simulink library "posAug_cl_old"  (R2022a)
settings: Solver=VariableStepAuto  StartTime=0.0  StopTime=10.0  RelTol=1e-3
undefined symbols (not defined in the file): aoaStart, elevSet, elevStart, env, FLIGHTCONTROLLER, fltCtrl, initializeBussesFromBlock, intSat, pathLaps, pathLapsYaw, posAug, rollAmp, rollFreq, rollPhase, sEstim, slfExitTime, thetaIGain, thetaPGain, vhcl, yawAmp, yawFreq, yawPhase
libraries: slpidlib x10, simulink x5, posAug_cl_new x4, velocityAngle_ul x4, dspsigops x3, pathFollowingCtrlAoATurb_cl x1, pathFollowingCtrlAoATurbCoef_cl x1, courseFollowLookAhead_cl x1, ctrlAllocMatrix3CompCoef_cl x1, eulAng2RotMat_ul x1, $bdroot x1, angleBtw2Vecs_ul x1
(part 3 of 3)

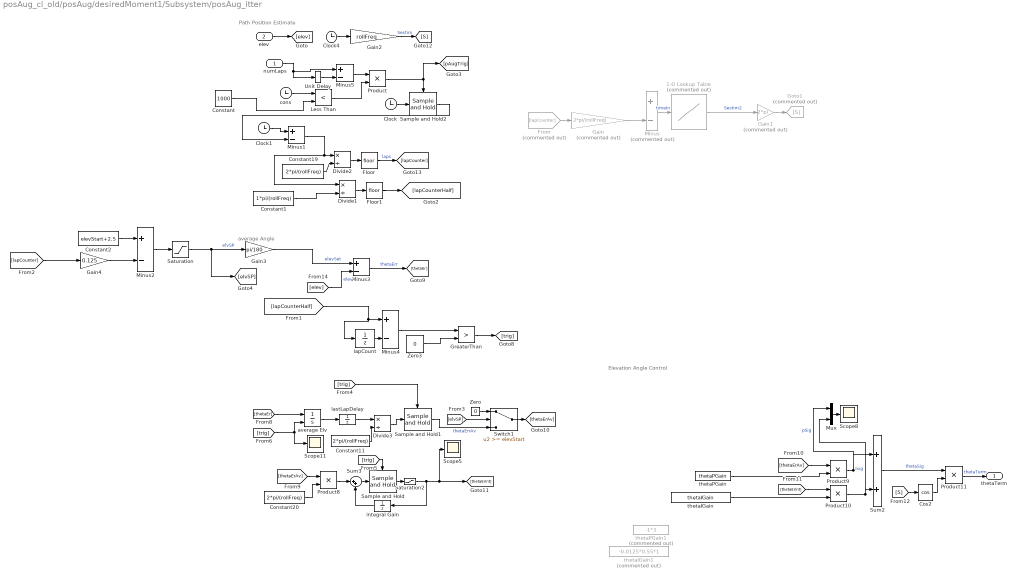
== system posAug_cl_old/posAug/desiredMoment1/Subsystem/posAug_itter ==
  note: average Angle
  note: Path Position Estimate
  note: Elevation Angle Control
  numLaps : Inport
  elev : Inport  Port=2
  1-D Lookup Table : Lookup_n-D  Commented=on  NumberOfTableDimensions=1  BreakpointsForDimension1=times  Table=sEstim  ExtrapMethod=Clip  InternalRulePriority=Speed  RndMeth=Simplest
  Clock : Clock
  Clock1 : Clock
  Clock4 : Clock
  Constant : Constant  Value=1000
  Constant1 : Constant  Value=1*pi/(rollFreq)
  Constant11 : Constant  Value=2*pi/(rollFreq)
  Constant19 : Constant  Value=2*pi/(rollFreq)
  Constant2 : Constant  Value=elevStart+2.5
  Constant20 : Constant  Value=2*pi/(rollFreq)
  Cos2 : Trigonometry  Operator=cos
  Divide1 : Product  Inputs=*/
  Divide2 : Product  Inputs=*/
  Divide3 : Product  Inputs=*/
  Floor : Rounding
  Floor1 : Rounding
  From : From  Commented=on  GotoTag=lapCounter
  Gain : Gain  Commented=on  Gain=2*pi/(rollFreq)
  Gain1 : Gain  Commented=on  Gain=2*pi
  Gain2 : Gain  Gain=rollFreq
  Gain3 : Gain  Gain=pi/180
  Gain4 : Gain  Gain=0.125
  Goto1 : Goto  Commented=on  GotoTag=S
  GreaterThan : RelationalOperator  Operator=>  OutDataTypeStr=boolean  RndMeth=Simplest  InputSameDT=off
  Less Than : RelationalOperator  Operator=<  OutDataTypeStr=boolean  RndMeth=Simplest  InputSameDT=off
  Minus : Sum  Commented=on  Inputs=+-
  Minus{1..5} (5 alike) : Sum  Inputs=+-
  Mux : Mux  Inputs=2
  Product{,8..11} (5 alike) : Product
  Sample and Hold : dspsigops/Sample and Hold  trig=Rising edge  initCond=0  latchinput=off
  Sample and Hold1 : dspsigops/Sample and Hold  trig=Rising edge  initCond=0  latchinput=off
  Sample and Hold2 : dspsigops/Sample and Hold  trig=Rising edge  initCond=0  latchinput=off
  Saturation : Saturate  UpperLimit=elevStart  LowerLimit=elevSet
  Saturation2 : Saturate  UpperLimit=intSat  LowerLimit=-intSat
  Scope11 : Scope
  Scope5 : Scope
  Scope8 : Scope
  Sum2 : Sum  Inputs=|++
  Sum3 : Sum  Inputs=|++
  Switch1 : Switch  Threshold=elevStart  SaturateOnIntegerOverflow=off  InputSameDT=off
  Unit Delay : UnitDelay  SampleTime=-1  HasFrameUpgradeWarning=on
  Zero : Constant  Value=0  OutDataTypeStr=Inherit: Inherit via back propagation
  Zero3 : Constant  Value=0  OutDataTypeStr=Inherit: Inherit via back propagation
  average Elv : Integrator  ExternalReset=rising
  cons : Clock
  integral Gain : UnitDelay  SampleTime=-1  HasFrameUpgradeWarning=on
  lapCount : UnitDelay  SampleTime=-1  HasFrameUpgradeWarning=on
  lastLapDelay : UnitDelay  SampleTime=-1  HasFrameUpgradeWarning=on
  thetaIGain : Constant  Value=thetaIGain
  thetaIGain1 : Constant  Commented=on  Value=-0.0125*0.55*1
  thetaPGain : Constant  Value=thetaPGain
  thetaPGain1 : Constant  Commented=on  Value=-1*3
  thetaTerm : Outport
  wires:
  Sum2/1 -> Product11/1  "thetaSig"
  [thetaErAv] -> Product8/1
  lapCount/1 -> Minus4/2
  thetaIGain/1 -> Product10/2
  Product11/1 -> thetaTerm/1  "thetaTerm"
  GreaterThan/1 -> [trig]
  thetaPGain/1 -> Product9/2
  [trig] -> Scope11/1, average Elv/2
  [thetaErInt] -> Product10/1
  [elev] -> Minus3/2  "elev"
  average Elv/1 -> lastLapDelay/1
  Divide2/1 -> Floor/1
  Zero3/1 -> GreaterThan/2
  Floor/1 -> [lapCounter]  "laps"
  [lapCounterHalf] -> lapCount/1, Minus4/1
  Product10/1 -> Mux/2, Sum2/2  "Isig"
  Mux/1 -> Scope8/1
  Product9/1 -> Mux/1, Sum2/1  "pSig"
  Cos2/1 -> Product11/2
  Saturation2/1 -> Scope5/1, [thetaErInt], integral Gain/1
  Sample and Hold1/1 -> Switch1/3  "thetaErrAv"
  Product8/1 -> Sum3/1
  [S] -> Cos2/1
  [trig] -> Sample and Hold1/Trigger
  [thetaErAv] -> Product9/1
  Constant20/1 -> Product8/2
  Sample and Hold/1 -> Saturation2/1
  integral Gain/1 -> Sum3/2
  Minus1/1 -> Divide1/1, Divide2/1
  Sample and Hold2/1 -> Minus1/2
  Divide3/1 -> Sample and Hold1/1
  Clock4/1 -> Gain2/1
  Saturation/1 -> [elvSP], Gain3/1  "elvSP"
  Constant11/1 -> Divide3/2
  Gain2/1 -> [S]  "Sestim"
  [trig] -> Sample and Hold/Trigger
  lastLapDelay/1 -> Divide3/1
  Minus3/1 -> [thetaEr]  "thetaErr"
  Minus4/1 -> GreaterThan/1
  [thetaEr] -> average Elv/1
  Sum3/1 -> Sample and Hold/1
  Constant19/1 -> Divide2/2
  Clock1/1 -> Minus1/1
  elev/1 -> [elev]
  Product/1 -> Sample and Hold2/Trigger, [pAugTrig]
  Clock/1 -> Sample and Hold2/1
  From/1 -> Gain/1
  Gain/1 -> Minus/2
  Minus/1 -> 1-D Lookup Table/1  "timeIn"
  1-D Lookup Table/1 -> Gain1/1  "Sestim2"
  Gain1/1 -> Goto1/1
  Divide1/1 -> Floor1/1
  Floor1/1 -> [lapCounterHalf]
  Constant1/1 -> Divide1/2
  [lapCounter] -> Gain4/1
  Constant2/1 -> Minus2/1
  Minus2/1 -> Saturation/1
  Gain3/1 -> Minus3/1  "elevSet"
  numLaps/1 -> Unit Delay/1, Minus5/1
  Unit Delay/1 -> Minus5/2
  [elvSP] -> Switch1/2
  Zero/1 -> Switch1/1
  Switch1/1 -> [thetaErAv]
  Gain4/1 -> Minus2/2
  Minus5/1 -> Product/1
  Less Than/1 -> Product/2
  cons/1 -> Less Than/1
  Constant/1 -> Less Than/2

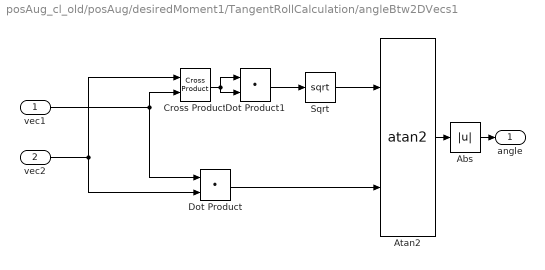
== system posAug_cl_old/posAug/desiredMoment1/TangentRollCalculation/angleBtw2DVecs1 ==
  vec1 : Inport
  vec2 : Inport  Port=2
  Abs : Abs  SaturateOnIntegerOverflow=off
  Atan2 : Trigonometry  Operator=atan2
  Cross Product : vrlib/Utilities/Cross Product
  Dot Product : DotProduct  OutDataTypeStr=Inherit: Inherit via internal rule
  Dot Product1 : DotProduct  OutDataTypeStr=Inherit: Inherit via internal rule
  Sqrt : Sqrt
  angle : Outport  VectorParamsAs1DForOutWhenUnconnected=off
  wires:
  Sqrt/1 -> Atan2/1
  Dot Product1/1 -> Sqrt/1
  Abs/1 -> angle/1
  Dot Product/1 -> Atan2/2
  Cross Product/1 -> Dot Product1/2, Dot Product1/1
  vec2/1 -> Dot Product/2, Cross Product/1
  vec1/1 -> Cross Product/2, Dot Product/1
  Atan2/1 -> Abs/1

== matlab function posAug_cl_old/posAug/desiredMoment1/MATLAB Function ==
  data: u input; y output
function y = fcn(u)

if abs(u)>2*pi

    y=sign(u)*(abs(u)-2*pi);
else
    y=u;
end
